simulink model "prelim_FFT"  (R2013a)
settings: Solver=ode45  StartTime=0.0  StopTime=10000  RelTol=1e-3
PostLoadFcn:
  | bps_model_init(gcs);
undefined symbols (not defined in the file or in its folder): xlipgetpartsetting
libraries: xbsIndex_r4 x75, xps_library x22, mbee4_library x4
(part 2 of 3)

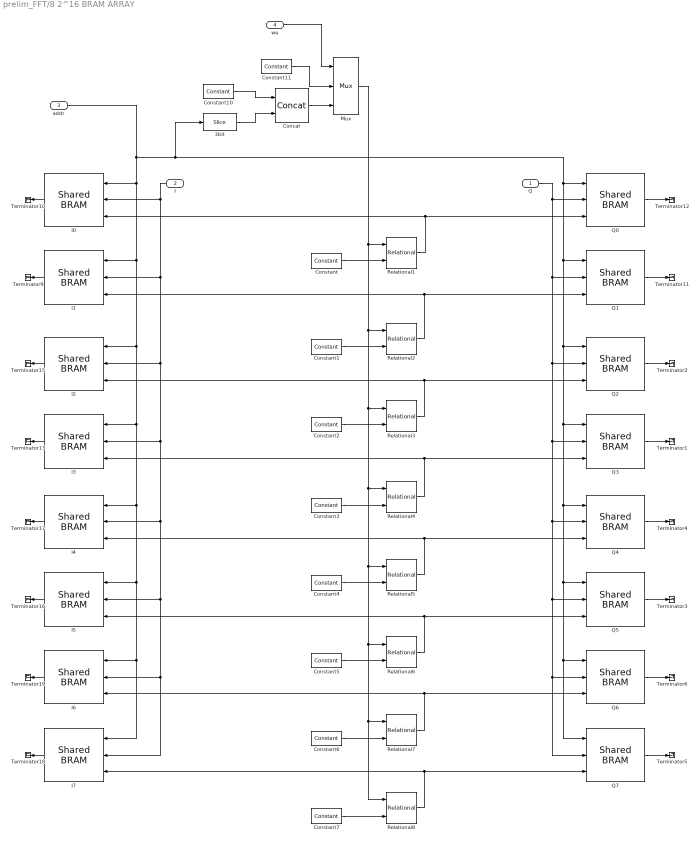
== system prelim_FFT/8 2^16 BRAM ARRAY ==
  Q : Inport
  I : Inport  Port=2
  addr : Inport  Port=3
  we : Inport  Port=4
  3bit : xbsIndex_r4/Slice  nbits=3  boolean_output=off  mode=Upper Bit Location + Width  bit1=0  base1=MSB of Input  bit0=0  base0=LSB of Input  dbl_ovrd=off  block_type=slice
  Concat : xbsIndex_r4/Concat  num_inputs=2  dbl_ovrd=off  block_type=concat
  Constant : xbsIndex_r4/Constant  const=0  gui_display_data_type=Fixed-point  arith_type=Unsigned  n_bits=4  bin_pt=0  preci_type=Single  exp_width=8  frac_width=24  explicit_period=off  period=1  equ=P=C  opselect=C  inp2=PCIN>>17  opr=+  inp1=P  carry=CIN  dbl_ovrd=off  block_type=constant
  Constant1 : xbsIndex_r4/Constant  const=1  gui_display_data_type=Fixed-point  arith_type=Unsigned  n_bits=4  bin_pt=0  preci_type=Single  exp_width=8  frac_width=24  explicit_period=off  period=1  equ=P=C  opselect=C  inp2=PCIN>>17  opr=+  inp1=P  carry=CIN  dbl_ovrd=off  block_type=constant
  Constant10 : xbsIndex_r4/Constant  const=0  gui_display_data_type=Fixed-point  arith_type=Unsigned  n_bits=3  bin_pt=0  preci_type=Single  exp_width=8  frac_width=24  explicit_period=off  period=1  equ=P=C  opselect=C  inp2=PCIN>>17  opr=+  inp1=P  carry=CIN  dbl_ovrd=off  block_type=constant
  Constant11 : xbsIndex_r4/Constant  const=15  gui_display_data_type=Fixed-point  arith_type=Unsigned  n_bits=4  bin_pt=0  preci_type=Single  exp_width=8  frac_width=24  explicit_period=off  period=1  equ=P=C  opselect=C  inp2=PCIN>>17  opr=+  inp1=P  carry=CIN  dbl_ovrd=off  block_type=constant
  Constant2 : xbsIndex_r4/Constant  const=2  gui_display_data_type=Fixed-point  arith_type=Unsigned  n_bits=4  bin_pt=0  preci_type=Single  exp_width=8  frac_width=24  explicit_period=off  period=1  equ=P=C  opselect=C  inp2=PCIN>>17  opr=+  inp1=P  carry=CIN  dbl_ovrd=off  block_type=constant
  Constant3 : xbsIndex_r4/Constant  const=3  gui_display_data_type=Fixed-point  arith_type=Unsigned  n_bits=4  bin_pt=0  preci_type=Single  exp_width=8  frac_width=24  explicit_period=off  period=1  equ=P=C  opselect=C  inp2=PCIN>>17  opr=+  inp1=P  carry=CIN  dbl_ovrd=off  block_type=constant
  Constant4 : xbsIndex_r4/Constant  const=4  gui_display_data_type=Fixed-point  arith_type=Unsigned  n_bits=4  bin_pt=0  preci_type=Single  exp_width=8  frac_width=24  explicit_period=off  period=1  equ=P=C  opselect=C  inp2=PCIN>>17  opr=+  inp1=P  carry=CIN  dbl_ovrd=off  block_type=constant
  Constant5 : xbsIndex_r4/Constant  const=5  gui_display_data_type=Fixed-point  arith_type=Unsigned  n_bits=4  bin_pt=0  preci_type=Single  exp_width=8  frac_width=24  explicit_period=off  period=1  equ=P=C  opselect=C  inp2=PCIN>>17  opr=+  inp1=P  carry=CIN  dbl_ovrd=off  block_type=constant
  Constant6 : xbsIndex_r4/Constant  const=6  gui_display_data_type=Fixed-point  arith_type=Unsigned  n_bits=4  bin_pt=0  preci_type=Single  exp_width=8  frac_width=24  explicit_period=off  period=1  equ=P=C  opselect=C  inp2=PCIN>>17  opr=+  inp1=P  carry=CIN  dbl_ovrd=off  block_type=constant
  Constant7 : xbsIndex_r4/Constant  const=7  gui_display_data_type=Fixed-point  arith_type=Unsigned  n_bits=4  bin_pt=0  preci_type=Single  exp_width=8  frac_width=24  explicit_period=off  period=1  equ=P=C  opselect=C  inp2=PCIN>>17  opr=+  inp1=P  carry=CIN  dbl_ovrd=off  block_type=constant
  I{0..7} (8 alike) : xps_library/Shared BRAM  Tag=xps:bram  arith_type=Unsigned  addr_width=16  bitwidth=32  bin_pt=0  init_vals=0  sample_period=1  update=off
  Mux : xbsIndex_r4/Mux  inputs=2  en=off  latency=0  precision=User Defined  arith_type=Unsigned  n_bits=4  bin_pt=0  quantization=Truncate  overflow=Wrap  dbl_ovrd=off  block_type=mux
  Q{0..7} (8 alike) : xps_library/Shared BRAM  Tag=xps:bram  arith_type=Unsigned  addr_width=16  bitwidth=32  bin_pt=0  init_vals=0  sample_period=1  update=off
  Relational{1..8} (8 alike) : xbsIndex_r4/Relational  mode=a=b  en=off  latency=0  dbl_ovrd=off  block_type=relational
  Terminator{1..6,9..13,15..19} (16 alike) : Terminator
  wires:
  Q/1 -> Q7/2, Q6/2, Q5/2, Q4/2, Q3/2, Q2/2, Q1/2, Q0/2
  addr/1 -> Q7/1, Q6/1, Q5/1, Q4/1, Q3/1, Q2/1, Q1/1, Q0/1, 3bit/1, I0/1, I1/1, I2/1, I3/1, I4/1, I6/1, I7/1, I5/1
  I/1 -> I1/2, I2/2, I3/2, I4/2, I5/2, I7/2, I6/2, I0/2
  Q1/1 -> Terminator11/1
  Q0/1 -> Terminator12/1
  Q3/1 -> Terminator1/1
  Q2/1 -> Terminator2/1
  Q5/1 -> Terminator3/1
  Q4/1 -> Terminator4/1
  Q7/1 -> Terminator5/1
  Q6/1 -> Terminator6/1
  I1/1 -> Terminator9/1
  I0/1 -> Terminator10/1
  I3/1 -> Terminator13/1
  I2/1 -> Terminator15/1
  I5/1 -> Terminator16/1
  I4/1 -> Terminator17/1
  I7/1 -> Terminator18/1
  I6/1 -> Terminator19/1
  we/1 -> Mux/1
  Constant/1 -> Relational1/2
  Constant1/1 -> Relational2/2
  Constant2/1 -> Relational3/2
  Constant3/1 -> Relational4/2
  Constant4/1 -> Relational5/2
  Constant5/1 -> Relational6/2
  Constant6/1 -> Relational7/2
  Constant7/1 -> Relational8/2
  Mux/1 -> Relational3/1, Relational4/1, Relational5/1, Relational7/1, Relational8/1, Relational6/1, Relational2/1, Relational1/1
  Relational1/1 -> Q0/3, I0/3
  Relational2/1 -> Q1/3, I1/3
  Relational3/1 -> I2/3, Q2/3
  Relational4/1 -> I3/3, Q3/3
  Relational5/1 -> I4/3, Q4/3
  Relational6/1 -> I5/3, Q5/3
  Relational7/1 -> I6/3, Q6/3
  Relational8/1 -> I7/3, Q7/3
  Concat/1 -> Mux/3
  3bit/1 -> Concat/2
  Constant10/1 -> Concat/1
  Constant11/1 -> Mux/2
